simulink model "Improved_version"  (Simulink 7.3)
settings: Solver=ode45  StartTime=0.0  StopTime=10.0  RelTol=1e-3
undefined symbols (not defined in the file or in its folder): x
libraries: powerlib x57, powerlib_extras x20
settings Model: Creator=me  LastModifiedBy=me

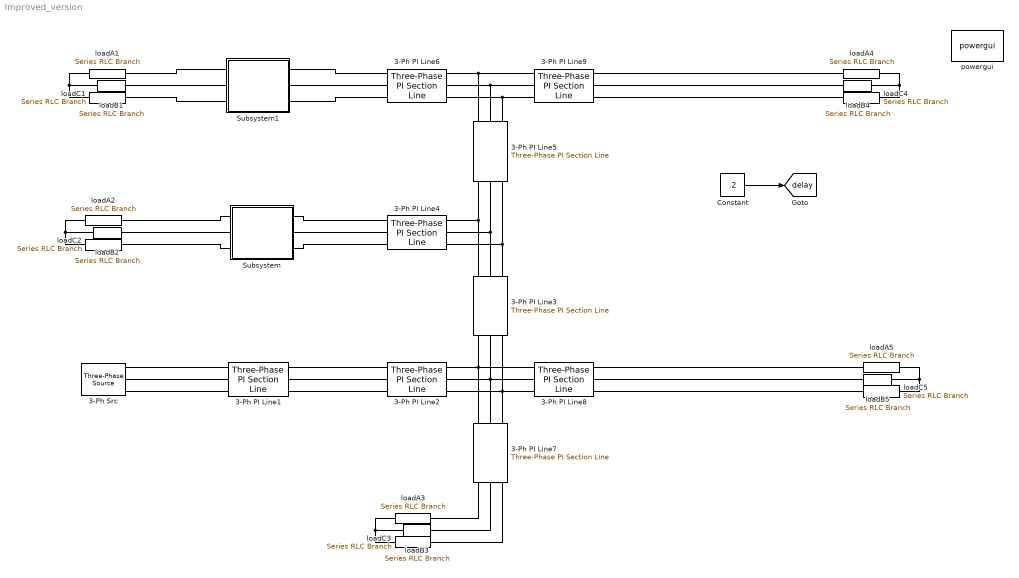
== system Improved_version ==
  3-Ph PI Line{1..9} (9 alike) : powerlib/Elements/Three-Phase PI Section Line  DialogController=POWERSYS.PowerSysDialog  PhysicalDomain=powersysdomain  SubClassName=unknown  LeftPortType=p1  RightPortType=p1  LConnTagsString=a|b|c  RConnTagsString=A|B|C  Frequency=60  Resistances=[ 0.01273 0.3864]  Inductances="[ 0.9337e-3  4.1264e-3]"  Capacitances=[12.74e-9 7.751e-9]  Length=100
  3-Ph Src : powerlib/Electrical Sources/Three-Phase Source  DialogController=POWERSYS.PowerSysDialog  SystemSampleTime=-1  Voltage=380  PhaseAngle=0  Frequency=50  InternalConnection=Yn  SpecifyImpedance=on  Resistance=0.8929  Inductance=16.58e-3  ShortCircuitLevel=100e6  BaseVoltage=380  XRratio=7
  Constant : Constant  Value=.2  OutDataType=fixdt(1, 16)  OutScaling=2^0
  Subsystem : Subsystem
  Subsystem1 : Subsystem
  loadA{1..5} (5 alike) : powerlib/Elements/Series RLC Branch  DialogController=POWERSYS.PowerSysDialog  PhysicalDomain=powersysdomain  SubClassName=unknown  LeftPortType=p1  RightPortType=p1  LConnTagsString=__new0  RConnTagsString=__new0  BranchType=Open circuit  Resistance=10  Inductance=30/(100*pi)  SetiL0=off  InitialCurrent=0  Capacitance=1/(100*pi)  Setx0=off  InitialVoltage=0  Measurements=None
  loadB{1..5} (5 alike) : powerlib/Elements/Series RLC Branch  DialogController=POWERSYS.PowerSysDialog  PhysicalDomain=powersysdomain  SubClassName=unknown  LeftPortType=p1  RightPortType=p1  LConnTagsString=__new0  RConnTagsString=__new0  BranchType=RC  Resistance=23  Inductance=50/(100*pi)  SetiL0=off  InitialCurrent=0  Capacitance=1/(1200*pi)  Setx0=off  InitialVoltage=0  Measurements=None
  loadC{1..5} (5 alike) : powerlib/Elements/Series RLC Branch  DialogController=POWERSYS.PowerSysDialog  PhysicalDomain=powersysdomain  SubClassName=unknown  LeftPortType=p1  RightPortType=p1  LConnTagsString=__new0  RConnTagsString=__new0  BranchType=RL  Resistance=14  Inductance=29/(100*pi)  SetiL0=off  InitialCurrent=0  Capacitance=1.0  Setx0=off  InitialVoltage=0  Measurements=None
  powergui : powerlib/powergui  Priority=1  SystemSampleTime=-1  SimulationMode=Continuous  SampleTime=50e-6  frequency=60  SPID=off  DisableSnubberDevices=off  DisableRonSwitches=off  DisableVfSwitches=off  SwTol=0  Interpol=off  frequencyindice=50  echomessages=off  HookPort=off  DisplayEquations=off  FunctionMessages=off  EnableUseOfTLC=off  x0status=blocks  RestoreLinks=warning  Frange=[0:2:500]  Ylog=off  Xlog=on  ShowGrid=off  save=off  variable=ZData  ZoomFFT=on  StartTime=0.0  cycles=1  DisplayStyle=1  fundamental=60  FreqAxis=off  MaxFrequency=1000  frequencyindicesteady=1  RmsSteady=1  display=off  Ts=0  methode=off
  tag scope: delay=global
  wires:
  Constant/1 -> [delay]
  connections:
  loadA1/RConn1 -- loadC1/RConn1 -- loadB1/RConn1
  loadB2/RConn1 -- loadA2/RConn1 -- loadC2/RConn1
  loadB3/RConn1 -- loadA3/RConn1 -- loadC3/RConn1
  loadA4/LConn1 -- loadC4/LConn1 -- loadB4/LConn1
  loadB5/LConn1 -- loadA5/LConn1 -- loadC5/LConn1
  3-Ph Src/RConn3 -- 3-Ph PI Line1/LConn3
  3-Ph Src/RConn2 -- 3-Ph PI Line1/LConn2
  3-Ph Src/RConn1 -- 3-Ph PI Line1/LConn1
  3-Ph PI Line1/RConn1 -- 3-Ph PI Line2/LConn1
  3-Ph PI Line1/RConn2 -- 3-Ph PI Line2/LConn2
  3-Ph PI Line1/RConn3 -- 3-Ph PI Line2/LConn3
  3-Ph PI Line2/RConn1 -- 3-Ph PI Line3/RConn1 -- 3-Ph PI Line7/LConn1 -- 3-Ph PI Line8/LConn1
  3-Ph PI Line3/RConn2 -- 3-Ph PI Line2/RConn2 -- 3-Ph PI Line7/LConn2 -- 3-Ph PI Line8/LConn2
  3-Ph PI Line3/RConn3 -- 3-Ph PI Line2/RConn3 -- 3-Ph PI Line7/LConn3 -- 3-Ph PI Line8/LConn3
  3-Ph PI Line7/RConn1 -- loadA3/LConn1
  3-Ph PI Line7/RConn2 -- loadB3/LConn1
  3-Ph PI Line7/RConn3 -- loadC3/LConn1
  3-Ph PI Line3/LConn1 -- 3-Ph PI Line5/RConn1 -- 3-Ph PI Line4/LConn1
  3-Ph PI Line5/RConn2 -- 3-Ph PI Line3/LConn2 -- 3-Ph PI Line4/LConn2
  3-Ph PI Line5/RConn3 -- 3-Ph PI Line3/LConn3 -- 3-Ph PI Line4/LConn3
  3-Ph PI Line5/LConn1 -- 3-Ph PI Line6/LConn1 -- 3-Ph PI Line9/RConn1
  3-Ph PI Line5/LConn2 -- 3-Ph PI Line6/LConn2 -- 3-Ph PI Line9/RConn2
  3-Ph PI Line5/LConn3 -- 3-Ph PI Line6/LConn3 -- 3-Ph PI Line9/RConn3
  3-Ph PI Line9/LConn1 -- loadA4/RConn1
  3-Ph PI Line8/RConn1 -- loadA5/RConn1
  3-Ph PI Line8/RConn2 -- loadB5/RConn1
  3-Ph PI Line8/RConn3 -- loadC5/RConn1
  3-Ph PI Line9/LConn2 -- loadB4/RConn1
  3-Ph PI Line9/LConn3 -- loadC4/RConn1
  Subsystem/RConn1 -- loadA2/LConn1
  Subsystem/RConn2 -- loadB2/LConn1
  Subsystem/RConn3 -- loadC2/LConn1
  Subsystem/LConn1 -- 3-Ph PI Line4/RConn1
  Subsystem/LConn2 -- 3-Ph PI Line4/RConn2
  Subsystem/LConn3 -- 3-Ph PI Line4/RConn3
  Subsystem1/LConn1 -- 3-Ph PI Line6/RConn1
  Subsystem1/LConn2 -- 3-Ph PI Line6/RConn2
  Subsystem1/LConn3 -- 3-Ph PI Line6/RConn3
  Subsystem1/RConn1 -- loadA1/LConn1
  Subsystem1/RConn2 -- loadB1/LConn1
  loadC1/LConn1 -- Subsystem1/RConn3

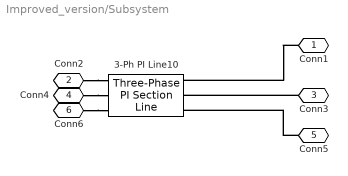
== system Improved_version/Subsystem ==
  3-Ph PI Line10 : powerlib/Elements/Three-Phase PI Section Line  DialogController=POWERSYS.PowerSysDialog  PhysicalDomain=powersysdomain  SubClassName=unknown  LeftPortType=p1  RightPortType=p1  LConnTagsString=a|b|c  RConnTagsString=A|B|C  Frequency=60  Resistances=[ 0.01273 0.3864]  Inductances="[ 0.9337e-3  4.1264e-3]"  Capacitances=[12.74e-9 7.751e-9]  Length=100
  Conn1 : PMIOPort  Port=1  Side=Left
  Conn2 : PMIOPort  Port=2  Side=Right
  Conn3 : PMIOPort  Port=3  Side=Left
  Conn4 : PMIOPort  Port=4  Side=Right
  Conn5 : PMIOPort  Port=5  Side=Left
  Conn6 : PMIOPort  Port=6  Side=Right
  connections:
  Conn1/RConn1 -- 3-Ph PI Line10/LConn1
  Conn2/RConn1 -- 3-Ph PI Line10/RConn1
  Conn3/RConn1 -- 3-Ph PI Line10/LConn2
  Conn4/RConn1 -- 3-Ph PI Line10/RConn2
  Conn5/RConn1 -- 3-Ph PI Line10/LConn3
  Conn6/RConn1 -- 3-Ph PI Line10/RConn3

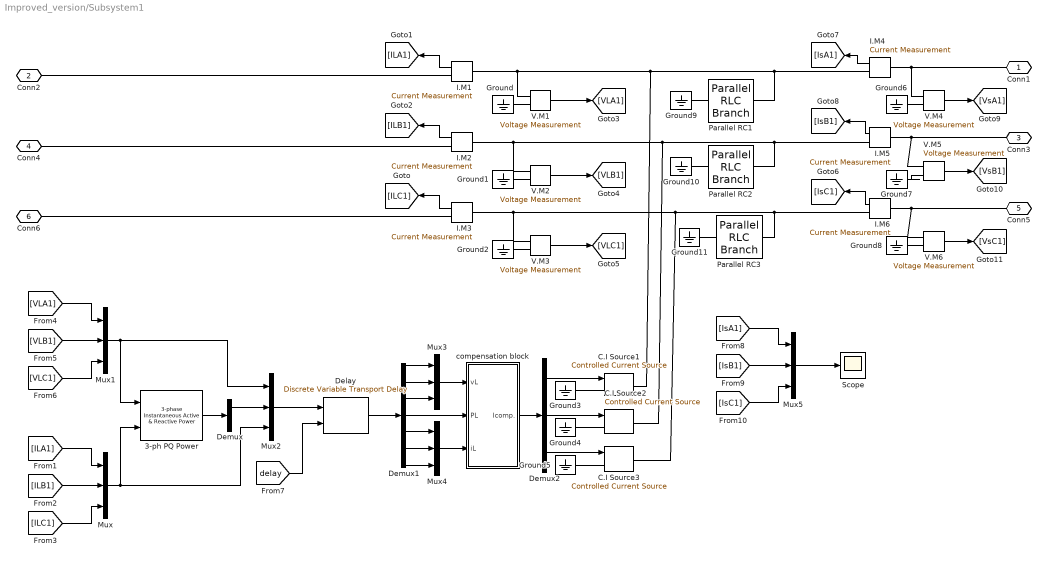
== system Improved_version/Subsystem1 ==
  3-ph PQ Power : powerlib_extras/Measurements/3-phase  Instantaneous  Active & Reactive Power  DialogController=POWERSYS.PowerSysDialog  SystemSampleTime=-1
  C.I Source1 : powerlib/Electrical Sources/Controlled Current Source  DialogController=POWERSYS.PowerSysDialog  SystemSampleTime=-1  Initialize=on  Source_Type=AC  Amplitude=0  Phase=0  Frequency=0  Measurements=None
  C.I Source2 : powerlib/Electrical Sources/Controlled Current Source  DialogController=POWERSYS.PowerSysDialog  SystemSampleTime=-1  Initialize=on  Source_Type=AC  Amplitude=0  Phase=0  Frequency=0  Measurements=None
  C.I Source3 : powerlib/Electrical Sources/Controlled Current Source  DialogController=POWERSYS.PowerSysDialog  SystemSampleTime=-1  Initialize=on  Source_Type=AC  Amplitude=0  Phase=0  Frequency=0  Measurements=None
  Delay : powerlib_extras/Discrete  Control Blocks/Discrete Variable Transport Delay  DialogController=POWERSYS.PowerSysDialog  SystemSampleTime=-1  MaxDelay=1/40  InitialValue=0  Ts=50e-6
  Demux : Demux  Outputs=2
  Demux1 : Demux  Outputs=7
  Demux2 : Demux  Outputs=3
  Ground{,1..11} (12 alike) : powerlib/Elements/Ground  DialogController=POWERSYS.PowerSysDialog  PhysicalDomain=powersysdomain  SubClassName=unknown  LeftPortType=p1  RightPortType=p1  LConnTagsString=a
  I.M{1..6} (6 alike) : powerlib/Measurements/Current Measurement  DialogController=POWERSYS.PowerSysDialog  SystemSampleTime=-1  PhasorSimulation=off  OutputType=Complex  PSBequivalent=0
  Mux{,1..5} (6 alike) : Mux  Inputs=3
  Parallel RC1 : powerlib/Elements/Parallel RLC Branch  DialogController=POWERSYS.PowerSysDialog  PhysicalDomain=powersysdomain  SubClassName=unknown  LeftPortType=p1  RightPortType=p1  LConnTagsString=a  RConnTagsString=__new0  BranchType=RC  Resistance=100  Inductance=1e-3  SetiL0=off  InitialCurrent=0  Capacitance=1/(10000*pi)  Setx0=off  InitialVoltage=0  Measurements=None
  Parallel RC2 : powerlib/Elements/Parallel RLC Branch  DialogController=POWERSYS.PowerSysDialog  PhysicalDomain=powersysdomain  SubClassName=unknown  LeftPortType=p1  RightPortType=p1  LConnTagsString=a  RConnTagsString=__new0  BranchType=RC  Resistance=100  Inductance=1e-3  SetiL0=off  InitialCurrent=0  Capacitance=1/(10000*pi)  Setx0=off  InitialVoltage=0  Measurements=None
  Parallel RC3 : powerlib/Elements/Parallel RLC Branch  DialogController=POWERSYS.PowerSysDialog  PhysicalDomain=powersysdomain  SubClassName=unknown  LeftPortType=p1  RightPortType=p1  LConnTagsString=a  RConnTagsString=__new0  BranchType=RC  Resistance=100  Inductance=1e-3  SetiL0=off  InitialCurrent=0  Capacitance=1/(10000*pi)  Setx0=off  InitialVoltage=0  Measurements=None
  Scope : Scope
      settings: TimeRange=0.5  YMin=-3  YMax=3
  V.M{1..6} (6 alike) : powerlib/Measurements/Voltage Measurement  DialogController=POWERSYS.PowerSysDialog  SystemSampleTime=-1  PhasorSimulation=off  OutputType=Complex  PSBequivalent=0
  compensation block : Subsystem
  Conn1 : PMIOPort  Port=1  Side=Left
  Conn2 : PMIOPort  Port=2  Side=Right
  Conn3 : PMIOPort  Port=3  Side=Left
  Conn4 : PMIOPort  Port=4  Side=Right
  Conn5 : PMIOPort  Port=5  Side=Left
  Conn6 : PMIOPort  Port=6  Side=Right
  wires:
  I.M1/1 -> [ILA1]
  I.M2/1 -> [ILB1]
  V.M1/1 -> [VLA1]
  V.M2/1 -> [VLB1]
  V.M3/1 -> [VLC1]
  [ILB1] -> Mux/2
  [ILA1] -> Mux/1
  [ILC1] -> Mux/3
  [VLB1] -> Mux1/2
  [VLA1] -> Mux1/1
  [VLC1] -> Mux1/3
  Mux1/1 -> 3-ph PQ Power/1, Mux2/1
  Mux/1 -> 3-ph PQ Power/2, Mux2/3
  3-ph PQ Power/1 -> Demux/1
  Demux/1 -> Mux2/2
  Mux2/1 -> Delay/1
  [delay] -> Delay/2
  Delay/1 -> Demux1/1
  Demux1/6 -> Mux4/2
  Demux1/5 -> Mux4/1
  Demux1/7 -> Mux4/3
  Demux1/1 -> Mux3/1
  Demux1/2 -> Mux3/2
  Demux1/3 -> Mux3/3
  Mux3/1 -> compensation block/1(vL)
  Demux1/4 -> compensation block/2(PL)
  Mux4/1 -> compensation block/3(iL)
  compensation block/1(Icomp.) -> Demux2/1
  Demux2/1 -> C.I Source1/1
  Demux2/2 -> C.I Source2/1
  Demux2/3 -> C.I Source3/1
  I.M3/1 -> [ILC1]
  I.M5/1 -> [IsB1]
  V.M4/1 -> [VsA1]
  V.M5/1 -> [VsB1]
  V.M6/1 -> [VsC1]
  I.M6/1 -> [IsC1]
  I.M4/1 -> [IsA1]
  [IsB1] -> Mux5/2
  [IsA1] -> Mux5/1
  [IsC1] -> Mux5/3
  Mux5/1 -> Scope/1
  connections:
  I.M4/RConn1 -- C.I Source1/RConn1 -- I.M1/LConn1 -- V.M1/LConn1 -- Parallel RC1/RConn1
  Conn2/RConn1 -- I.M1/RConn1
  I.M5/RConn1 -- C.I Source2/RConn1 -- I.M2/LConn1 -- V.M2/LConn1 -- Parallel RC2/RConn1
  Conn4/RConn1 -- I.M2/RConn1
  I.M6/RConn1 -- C.I Source3/RConn1 -- I.M3/LConn1 -- V.M3/LConn1 -- Parallel RC3/RConn1
  Ground/LConn1 -- V.M1/LConn2
  Ground1/LConn1 -- V.M2/LConn2
  Ground2/LConn1 -- V.M3/LConn2
  Ground5/LConn1 -- C.I Source3/LConn1
  Ground4/LConn1 -- C.I Source2/LConn1
  Ground3/LConn1 -- C.I Source1/LConn1
  Conn6/RConn1 -- I.M3/RConn1
  Conn1/RConn1 -- V.M4/LConn1 -- I.M4/LConn1
  V.M5/LConn1 -- I.M5/LConn1 -- Conn3/RConn1
  V.M6/LConn1 -- I.M6/LConn1 -- Conn5/RConn1
  Ground6/LConn1 -- V.M4/LConn2
  Ground7/LConn1 -- V.M5/LConn2
  Ground8/LConn1 -- V.M6/LConn2
  Parallel RC3/LConn1 -- Ground11/LConn1
  Parallel RC2/LConn1 -- Ground10/LConn1
  Parallel RC1/LConn1 -- Ground9/LConn1

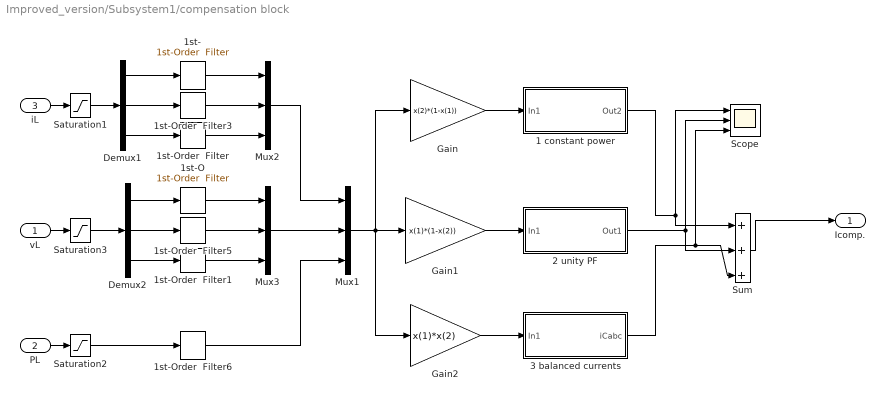
== system Improved_version/Subsystem1/compensation block ==
  vL : Inport  OutDataType=fixdt(1, 16)  OutScaling=2^0
  PL : Inport  Port=2  OutDataType=fixdt(1, 16)  OutScaling=2^0
  iL : Inport  Port=3  OutDataType=fixdt(1, 16)  OutScaling=2^0
  1 constant power : Subsystem
  1st- : powerlib_extras/Control  Blocks/1st-Order  Filter  DialogController=POWERSYS.PowerSysDialog  SystemSampleTime=-1  FilterType=Lowpass  Tc=.00051  Initialize=off  Vac_Init=[0.8 -25 60]  Vdc_Init=-0.4  PlotResponse=off  param1=[1 500 1]
  1st-O : powerlib_extras/Control  Blocks/1st-Order  Filter  DialogController=POWERSYS.PowerSysDialog  SystemSampleTime=-1  FilterType=Lowpass  Tc=.00051  Initialize=off  Vac_Init=[0.8 -25 60]  Vdc_Init=-0.4  PlotResponse=off  param1=[1 500 1]
  1st-Order  Filter{,1,3,5..6} (5 alike) : powerlib_extras/Control  Blocks/1st-Order  Filter  DialogController=POWERSYS.PowerSysDialog  SystemSampleTime=-1  FilterType=Lowpass  Tc=.00051  Initialize=off  Vac_Init=[0.8 -25 60]  Vdc_Init=-0.4  PlotResponse=off  param1=[1 500 1]
  2 unity PF : Subsystem
  "3 balanced currents " : Subsystem
  Demux1 : Demux  Outputs=3
  Demux2 : Demux  Outputs=3
  Gain : Gain  Gain=x(2)*(1-x(1))  ParameterDataType=fixdt(1, 16)  ParameterScaling=2^0  OutDataType=fixdt(1, 16)  OutScaling=2^0
  Gain1 : Gain  Gain=x(1)*(1-x(2))  ParameterDataType=fixdt(1, 16)  ParameterScaling=2^0  OutDataType=fixdt(1, 16)  OutScaling=2^0
  Gain2 : Gain  Gain=x(1)*x(2)  ParameterDataType=fixdt(1, 16)  ParameterScaling=2^0  OutDataType=fixdt(1, 16)  OutScaling=2^0
  Mux1 : Mux  Inputs=3
  Mux2 : Mux  Inputs=3
  Mux3 : Mux  Inputs=3
  Saturation1 : Saturate  UpperLimit=100  LowerLimit=-100  OutDataType=sfix(16)  OutScaling=2^0
  Saturation2 : Saturate  UpperLimit=10000  LowerLimit=0  OutDataType=sfix(16)  OutScaling=2^0
  Saturation3 : Saturate  UpperLimit=500  LowerLimit=-500  OutDataType=sfix(16)  OutScaling=2^0
  Scope : Scope  NumInputPorts=3
      settings: YMin=-7.5~-1~-1  YMax=10~1~1  SaveName=ScopeData33
  Sum : Sum  Inputs=|+++  OutDataType=fixdt(1, 16)  OutScaling=2^0
  Icomp. : Outport  OutDataType=sfix(16)  OutScaling=2^0
  wires:
  vL/1 -> Saturation3/1
  Demux1/1 -> 1st-/1
  Demux1/2 -> 1st-Order  Filter3/1
  Demux1/3 -> 1st-Order  Filter/1
  Saturation1/1 -> Demux1/1
  1st-Order  Filter1/1 -> Mux3/3
  Demux2/1 -> 1st-O/1
  Demux2/2 -> 1st-Order  Filter5/1
  Demux2/3 -> 1st-Order  Filter1/1
  1st-O/1 -> Mux3/1
  1st-Order  Filter5/1 -> Mux3/2
  Saturation2/1 -> 1st-Order  Filter6/1
  1st-/1 -> Mux2/1
  1st-Order  Filter3/1 -> Mux2/2
  1st-Order  Filter/1 -> Mux2/3
  Saturation3/1 -> Demux2/1
  iL/1 -> Saturation1/1
  PL/1 -> Saturation2/1
  Mux3/1 -> Mux1/2
  Mux2/1 -> Mux1/1
  1st-Order  Filter6/1 -> Mux1/3
  Gain/1 -> 1 constant power/1(In1)
  Mux1/1 -> Gain/1, Gain1/1, Gain2/1
  Gain1/1 -> 2 unity PF/1(In1)
  1 constant power/1(Out2) -> Sum/1, Scope/1
  2 unity PF/1(Out1) -> Sum/2, Scope/2
  Gain2/1 -> "3 balanced currents "/1(In1)
  "3 balanced currents "/1(iCabc) -> Sum/3, Scope/3
  Sum/1 -> Icomp./1

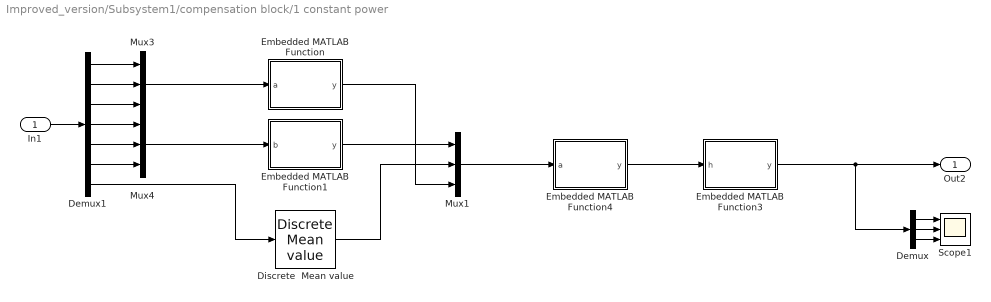
== system Improved_version/Subsystem1/compensation block/1 constant power ==
  In1 : Inport  OutDataType=fixdt(1, 16)  OutScaling=2^0
  Demux : Demux  Outputs=3
  Demux1 : Demux  Outputs=7
  Discrete  Mean value : powerlib_extras/Discrete Measurements/Discrete  Mean value  DialogController=POWERSYS.PowerSysDialog  SystemSampleTime=-1  Freq=50  Vinit=.001  Ts=50e-6
  Embedded MATLAB Function : Stateflow chart  TreatAsAtomicUnit=on
  Embedded MATLAB Function1 : Stateflow chart  TreatAsAtomicUnit=on
  Embedded MATLAB Function3 : Stateflow chart  TreatAsAtomicUnit=on
  Embedded MATLAB Function4 : Stateflow chart  TreatAsAtomicUnit=on
  Mux1 : Mux  Inputs=3
  Mux3 : Mux  Inputs=3
  Mux4 : Mux  Inputs=3
  Scope1 : Scope  NumInputPorts=3
      settings: YMin=-1~-1~-1  YMax=1~1~1  SaveName=ScopeData32
  Out2 : Outport  OutDataType=sfix(16)  OutScaling=2^0
  wires:
  Mux3/1 -> Embedded MATLAB Function/1(a)
  Mux4/1 -> Embedded MATLAB Function1/1(b)
  Embedded MATLAB Function3/1(y) -> Demux/1, Out2/1
  Embedded MATLAB Function4/1(y) -> Embedded MATLAB Function3/1(h)
  Mux1/1 -> Embedded MATLAB Function4/1(a)
  Discrete  Mean value/1 -> Mux1/2
  Embedded MATLAB Function1/1(y) -> Mux1/1
  Demux/3 -> Scope1/3
  Demux/2 -> Scope1/2
  Demux/1 -> Scope1/1
  Embedded MATLAB Function/1(y) -> Mux1/3
  In1/1 -> Demux1/1
  Demux1/1 -> Mux3/1
  Demux1/2 -> Mux3/2
  Demux1/3 -> Mux3/3
  Demux1/4 -> Mux4/1
  Demux1/5 -> Mux4/2
  Demux1/6 -> Mux4/3
  Demux1/7 -> Discrete  Mean value/1

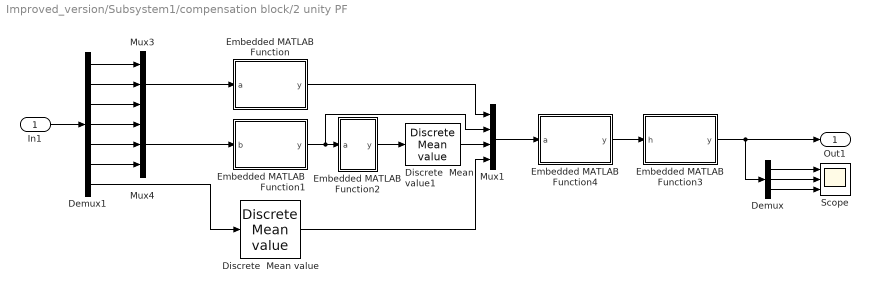
== system Improved_version/Subsystem1/compensation block/2 unity PF ==
  In1 : Inport  OutDataType=fixdt(1, 16)  OutScaling=2^0
  Demux : Demux  Outputs=3
  Demux1 : Demux  Outputs=7
  Discrete  Mean value : powerlib_extras/Discrete Measurements/Discrete  Mean value  DialogController=POWERSYS.PowerSysDialog  SystemSampleTime=-1  Freq=50  Vinit=0  Ts=50e-6
  Discrete  Mean value1 : powerlib_extras/Discrete Measurements/Discrete  Mean value  DialogController=POWERSYS.PowerSysDialog  SystemSampleTime=-1  Freq=50  Vinit=0  Ts=50e-6
  Embedded MATLAB Function : Stateflow chart  TreatAsAtomicUnit=on
  Embedded MATLAB Function1 : Stateflow chart  TreatAsAtomicUnit=on
  Embedded MATLAB Function2 : Stateflow chart  TreatAsAtomicUnit=on
  Embedded MATLAB Function3 : Stateflow chart  TreatAsAtomicUnit=on
  Embedded MATLAB Function4 : Stateflow chart  TreatAsAtomicUnit=on
  Mux1 : Mux
  Mux3 : Mux  Inputs=3
  Mux4 : Mux  Inputs=3
  Scope : Scope  NumInputPorts=3
      settings: YMin=-1~-1~-1  YMax=1~1~1  SaveName=ScopeData31
  Out1 : Outport  OutDataType=sfix(16)  OutScaling=2^0
  wires:
  Embedded MATLAB Function1/1(y) -> Embedded MATLAB Function2/1(a), Mux1/2
  Demux1/7 -> Discrete  Mean value/1
  Mux4/1 -> Embedded MATLAB Function1/1(b)
  Mux3/1 -> Embedded MATLAB Function/1(a)
  Demux1/6 -> Mux4/3
  Demux1/5 -> Mux4/2
  Demux1/4 -> Mux4/1
  Demux1/3 -> Mux3/3
  Demux1/2 -> Mux3/2
  Demux1/1 -> Mux3/1
  In1/1 -> Demux1/1
  Embedded MATLAB Function/1(y) -> Mux1/1
  Discrete  Mean value1/1 -> Mux1/3
  Embedded MATLAB Function2/1(y) -> Discrete  Mean value1/1
  Embedded MATLAB Function3/1(y) -> Out1/1, Demux/1
  Embedded MATLAB Function4/1(y) -> Embedded MATLAB Function3/1(h)
  Mux1/1 -> Embedded MATLAB Function4/1(a)
  Discrete  Mean value/1 -> Mux1/4
  Demux/3 -> Scope/3
  Demux/2 -> Scope/2
  Demux/1 -> Scope/1

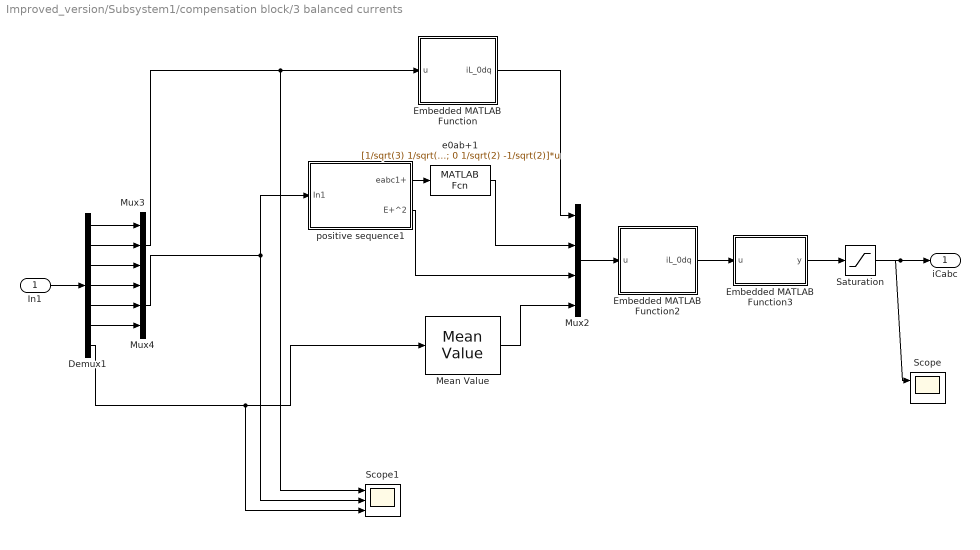
== system Improved_version/Subsystem1/compensation block/3 balanced currents  ==
  In1 : Inport  OutDataType=fixdt(1, 16)  OutScaling=2^0
  Demux1 : Demux  Outputs=7
  Embedded MATLAB Function : Stateflow chart  TreatAsAtomicUnit=on
  Embedded MATLAB Function2 : Stateflow chart  TreatAsAtomicUnit=on
  Embedded MATLAB Function3 : Stateflow chart  TreatAsAtomicUnit=on
  Mean Value : powerlib_extras/Measurements/Mean Value  DialogController=POWERSYS.PowerSysDialog  SystemSampleTime=-1  Period=1/60
  Mux2 : Mux
  Mux3 : Mux  Inputs=3
  Mux4 : Mux  Inputs=3
  Saturation : Saturate  UpperLimit=100  LowerLimit=-100  OutDataType=sfix(16)  OutScaling=2^0
  Scope : Scope  NumInputPorts=2
      settings: YMin=-200~-1  YMax=200~1  SaveName=ScopeData34
  Scope1 : Scope  NumInputPorts=3
      settings: YMin=-30~-500~0  YMax=25~500~7000  SaveName=ScopeData35
  e0ab+1 : MATLABFcn  MATLABFcn=[1/sqrt(3) 1/sqrt(3) 1/sqrt(3); sqrt(2)/sqrt(3) -1/sqrt(6) -1/sqrt(6); 0 1/sqrt(2) -1/sqrt(2)]*u
  positive sequence1 : Subsystem
  iCabc : Outport  OutDataType=fixdt(1, 16)  OutScaling=2^0
  wires:
  In1/1 -> Demux1/1
  Demux1/1 -> Mux3/1
  Demux1/2 -> Mux3/2
  Demux1/3 -> Mux3/3
  Demux1/4 -> Mux4/1
  Demux1/5 -> Mux4/2
  Demux1/6 -> Mux4/3
  Embedded MATLAB Function/1(iL_0dq) -> Mux2/1
  e0ab+1/1 -> Mux2/2
  Mean Value/1 -> Mux2/4
  Mux2/1 -> Embedded MATLAB Function2/1(u)
  Embedded MATLAB Function2/1(iL_0dq) -> Embedded MATLAB Function3/1(u)
  Embedded MATLAB Function3/1(y) -> Saturation/1
  positive sequence1/2(E+^2) -> Mux2/3
  positive sequence1/1(eabc1+) -> e0ab+1/1
  Saturation/1 -> iCabc/1, Scope/1
  Mux3/1 -> Embedded MATLAB Function/1(u), Scope1/1
  Mux4/1 -> positive sequence1/1(In1), Scope1/2
  Demux1/7 -> Mean Value/1, Scope1/3

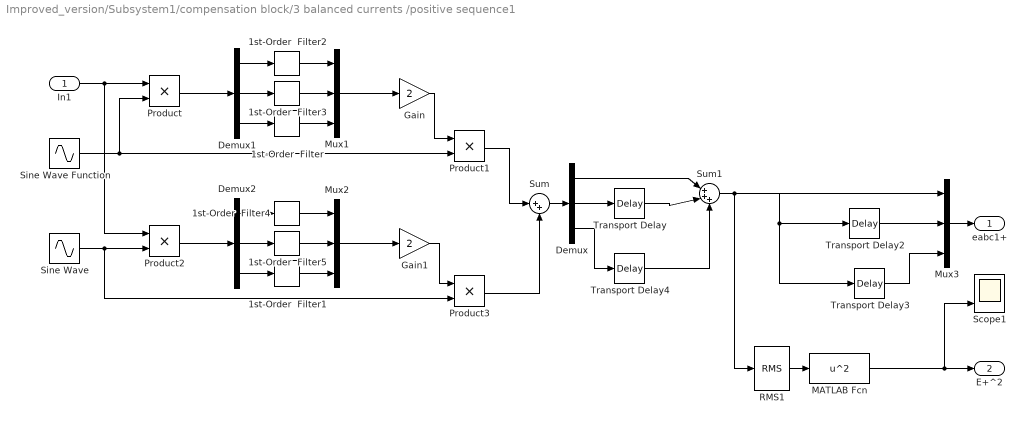
== system Improved_version/Subsystem1/compensation block/3 balanced currents /positive sequence1 ==
  In1 : Inport  OutDataType=sfix(16)  OutScaling=2^0
  1st-Order  Filter{,1,3,5} (4 alike) : powerlib_extras/Control  Blocks/1st-Order  Filter  DialogController=POWERSYS.PowerSysDialog  SystemSampleTime=-1  FilterType=Lowpass  Tc=.01  Initialize=off  Vac_Init=[0.8 -25 60]  Vdc_Init=-0.4  PlotResponse=off  param1=[1 500 1]
  1st-Order  Filter2 : powerlib_extras/Control  Blocks/1st-Order  Filter  DialogController=POWERSYS.PowerSysDialog  SystemSampleTime=-1  FilterType=Lowpass  Tc=.015  Initialize=off  Vac_Init=[0.8 -25 60]  Vdc_Init=-0.4  PlotResponse=off  param1=[1 500 1]
  1st-Order  Filter4 : powerlib_extras/Control  Blocks/1st-Order  Filter  DialogController=POWERSYS.PowerSysDialog  SystemSampleTime=-1  FilterType=Lowpass  Tc=.015  Initialize=off  Vac_Init=[0.8 -25 60]  Vdc_Init=-0.4  PlotResponse=off  param1=[1 500 1]
  Demux : Demux  Outputs=3
  Demux1 : Demux  Outputs=3
  Demux2 : Demux  Outputs=3
  Gain : Gain  Gain=2  ParameterDataType=sfix(16)  ParameterScaling=2^0  OutDataType=sfix(16)  OutScaling=2^0
  Gain1 : Gain  Gain=2  ParameterDataType=sfix(16)  ParameterScaling=2^0  OutDataType=sfix(16)  OutScaling=2^0
  MATLAB Fcn : MATLABFcn  MATLABFcn=u^2
  Mux1 : Mux  Inputs=3
  Mux2 : Mux  Inputs=3
  Mux3 : Mux  Inputs=3
  Product{,1..3} (4 alike) : Product  OutDataType=sfix(16)  OutScaling=2^0  RndMeth=Zero
  RMS1 : powerlib_extras/Measurements/RMS  DialogController=POWERSYS.PowerSysDialog  SystemSampleTime=-1  f1=50
  Scope1 : Scope  NumInputPorts=3
      settings: YMin=-1~-1~150000  YMax=1~1~320000
  Sine Wave : Sin  Amplitude=1  Bias=0  Frequency=100*pi  Phase=pi/2  Samples=10  SampleTime=0  Offset=0
  Sine Wave Function : Sin  Amplitude=1  Bias=0  Frequency=100*pi  Phase=0  Samples=10  SampleTime=0  Offset=0
  Sum : Sum  Inputs=|++  OutDataType=sfix(16)  OutScaling=2^0
  Sum1 : Sum  Inputs=|+++  OutDataType=sfix(16)  OutScaling=2^0
  Transport Delay : TransportDelay  DelayTime=.04/3
  Transport Delay2 : TransportDelay  DelayTime=.02/3
  Transport Delay3 : TransportDelay  DelayTime=.04/3
  Transport Delay4 : TransportDelay  DelayTime=.02/3
  eabc1+ : Outport  OutDataType=sfix(16)  OutScaling=2^0
  E+^2 : Outport  Port=2  OutDataType=sfix(16)  OutScaling=2^0
  wires:
  RMS1/1 -> MATLAB Fcn/1
  MATLAB Fcn/1 -> E+^2/1, Scope1/3
  In1/1 -> Product/1, Product2/1
  Sine Wave Function/1 -> Product/2, Product1/2
  1st-Order  Filter/1 -> Mux1/3
  Gain/1 -> Product1/1
  Sine Wave/1 -> Product2/2, Product3/2
  Gain1/1 -> Product3/1
  Product1/1 -> Sum/1
  Product3/1 -> Sum/2
  Sum/1 -> Demux/1
  Demux/2 -> Transport Delay/1
  Sum1/1 -> Transport Delay3/1, Mux3/1, RMS1/1, Transport Delay2/1
  Demux/3 -> Transport Delay4/1
  Transport Delay2/1 -> Mux3/2
  Transport Delay3/1 -> Mux3/3
  Mux3/1 -> eabc1+/1
  Demux1/1 -> 1st-Order  Filter2/1
  Demux1/2 -> 1st-Order  Filter3/1
  Demux1/3 -> 1st-Order  Filter/1
  Product/1 -> Demux1/1
  1st-Order  Filter2/1 -> Mux1/1
  1st-Order  Filter3/1 -> Mux1/2
  Mux1/1 -> Gain/1
  1st-Order  Filter1/1 -> Mux2/3
  Demux2/1 -> 1st-Order  Filter4/1
  Demux2/2 -> 1st-Order  Filter5/1
  Demux2/3 -> 1st-Order  Filter1/1
  Product2/1 -> Demux2/1
  1st-Order  Filter4/1 -> Mux2/1
  1st-Order  Filter5/1 -> Mux2/2
  Mux2/1 -> Gain1/1
  Demux/1 -> Sum1/1
  Transport Delay/1 -> Sum1/2
  Transport Delay4/1 -> Sum1/3

== matlab function Subsystem1/compensation block/1 constant power/Embedded MATLAB Function ==
  data: a input double; y output double
function y = fcn(a)
%#eml

y =[1/sqrt(3) 1/sqrt(3) 1/sqrt(3); sqrt(2)/sqrt(3) -sqrt(2)/(2*sqrt(3)) -sqrt(2)/(2*sqrt(3)); 0 1/sqrt(2) -1/sqrt(2)]*a;

== matlab function Subsystem1/compensation block/1 constant power/Embedded MATLAB Function1 ==
  data: b input double; y output double
function y = fcn(b)
%#eml

y = [1/sqrt(3) 1/sqrt(3) 1/sqrt(3); sqrt(2)/sqrt(3) -sqrt(2)/(2*sqrt(3)) -sqrt(2)/(2*sqrt(3)); 0 1/sqrt(2) -1/sqrt(2)]*b;

== matlab function Subsystem1/compensation block/1 constant power/Embedded MATLAB Function3 ==
  data: h input double; y output double
function y = fcn(h)
%#eml

y =[1/sqrt(3) sqrt(2)/sqrt(3) 0 ;1/sqrt(3) -sqrt(2)/(2*sqrt(3)) 1/sqrt(2) ;1/sqrt(3) -sqrt(2)/(2*sqrt(3)) -1/sqrt(2)]*h;

== matlab function Subsystem1/compensation block/1 constant power/Embedded MATLAB Function4 ==
  data: a input double; y output double
function y = fcn(a)
% #eml
if (a(2)^2+a(3)^2)==0
    y=[0; 0;0];
else
y =-[0;a(2);a(3)]*(a(4)/(a(2)^2+a(3)^2))+[a(5);a(6);a(7)];
end

== matlab function Subsystem1/compensation block/2 unity PF/Embedded MATLAB Function ==
  data: a input double; y output double
function y = fcn(a)
%#eml

y =[1/sqrt(3) 1/sqrt(3) 1/sqrt(3); sqrt(2)/sqrt(3) -sqrt(2)/(2*sqrt(3)) -sqrt(2)/(2*sqrt(3)); 0 1/sqrt(2) -1/sqrt(2)]*a;

== matlab function Subsystem1/compensation block/2 unity PF/Embedded MATLAB Function1 ==
  data: b input double; y output double
function y = fcn(b)
%#eml

y = [1/sqrt(3) 1/sqrt(3) 1/sqrt(3); sqrt(2)/sqrt(3) -sqrt(2)/(2*sqrt(3)) -sqrt(2)/(2*sqrt(3)); 0 1/sqrt(2) -1/sqrt(2)]*b;

== matlab function Subsystem1/compensation block/2 unity PF/Embedded MATLAB Function2 ==
  data: a input double; y output double
function y = fcn(a)
% #eml

y =(a(1)^2+a(2)^2+a(3)^2);

== matlab function Subsystem1/compensation block/2 unity PF/Embedded MATLAB Function3 ==
  data: h input double; y output double
function y = fcn(h)
%#eml

y =[1/sqrt(3) sqrt(2)/sqrt(3) 0 ;1/sqrt(3) -sqrt(2)/(2*sqrt(3)) 1/sqrt(2) ;1/sqrt(3) -sqrt(2)/(2*sqrt(3)) -1/sqrt(2)]*h;

== matlab function Subsystem1/compensation block/2 unity PF/Embedded MATLAB Function4 ==
  data: a input double; y output double
function y = fcn(a)
% #eml
if a(7)<10
    y=[0; 0;0];
else
y =[a(1);a(2);a(3)]-[a(4);a(5);a(6)]*((a(8)/a(7)));
end

== matlab function Subsystem1/compensation block/3 balanced currents /Embedded MATLAB Function ==
  data: u input double; iL_0dq output double
function iL_0dq = fcn(u)
%#eml

iL_0dq =[1/sqrt(3) 1/sqrt(3) 1/sqrt(3); sqrt(2)/sqrt(3) -sqrt(2)/(2*sqrt(3)) -sqrt(2)/(2*sqrt(3)); 0 1/sqrt(2) -1/sqrt(2)]*u;

== matlab function Subsystem1/compensation block/3 balanced currents /Embedded MATLAB Function2 ==
  data: u input double; iL_0dq output double
function iL_0dq = fcn(u)
%#eml
if u(7)==0
    iL_0dq=[0;0;0];
else
iL_0dq =[u(1);u(2);u(3)]-(u(8)/u(7))*[0;u(5);u(6)];
end

== matlab function Subsystem1/compensation block/3 balanced currents /Embedded MATLAB Function3 ==
  data: u input double; y output double
function y = fcn(u)
%#eml

y =[1/sqrt(3) sqrt(2)/sqrt(3) 0 ;1/sqrt(3) -sqrt(2)/(2*sqrt(3)) 1/sqrt(2) ;1/sqrt(3) -sqrt(2)/(2*sqrt(3)) -1/sqrt(2)]*u;
